simulink model "EEE3099S_Group12_Maze_Sim"  (R2021b)
settings: Solver=FixedStepDiscrete  StartTime=0.0  StopTime=20  FixedStep=0.01  RelTol=1e-3
values from neighbouring files (symbols this model uses):
  axleLength = 0.136    [robotParameters.m]    (also in straight_line.mat = 0.28)
  InputPWM = [-127 -126 -125 -124 -123 -122 -121 -120 -119 -118 -117 -116 ... (173 elements, 1x173)]    [straight_line.mat]
  ticksPerRot = 20    [robotParameters.m]    (also in straight_line.mat)
  wheelR = 0.031    [robotParameters.m]    (also in straight_line.mat = 0.052)
  WheelSpeed = [-12.5105278523 -12.3751973908 -12.2398669292 -12.1045364677 -11.9692060062 -11.8338755446 -11.6985450831 -11.5632146215 -11.42788416 -11.2925536985 -11.1572232369 -11.0218927754 ... (173 elements, 1x173)]    [straight_line.mat]
libraries: mobileRoboticsTrainingLib x6, slpidlib x1, simulink_extras x1
settings Model: ExtModeTrigDuration=2  Creator=Boitumelo  LastModifiedBy=ryanj
settings OptimizationCC: EnhancedBackFolding=on  PassReuseOutputArgsAs=Individual arguments  ZeroExternalMemoryAtStartup=off  ZeroInternalMemoryAtStartup=off  MaxStackSize=64  OptimizeBlockOrder=speed  DifferentSizesBufferReuse=on  OptimizationCustomize=off  EfficientTunableParamExpr=on
settings DebuggingCC: ParameterTunabilityLossMsg=error
settings HardwareCC: ProdBitPerPointer=32  ProdBitPerSizeT=32  ProdBitPerPtrDiffT=32  ProdLargestAtomicInteger=Long  ProdLargestAtomicFloat=Double  ProdWordSize=32  ProdHWDeviceType=ARM Compatible->ARM Cortex  UseEmbeddedCoderFeatures=off  UseSimulinkCoderFeatures=off
settings SFSimCC: MATLABDynamicMemAlloc=off
settings RTWCC: Description=Embedded Coder  SystemTargetFile=ert.tlc  HardwareBoard=Arduino Nano 33 IoT  TemplateMakefile=ert_default_tmf  Toolchain=Arduino ARM
settings CodeAppCC: ForceParamTrailComments=on  IgnoreCustomStorageClasses=off  OperatorAnnotations=on  SimulinkDataObjDesc=on  SFDataObjDesc=on  InsertBlockDesc=on
settings ERTTargetCC: SupportContinuousTime=on  SupportNonInlinedSFcns=on  SupportVariableSizeSignals=on  ExtModeTransport=3  ExtModeStaticAlloc=on  ExtModeStaticAllocSize=8192  ExtModeMexFile=ext_xcp  ExtModeIntrfLevel=Level2 - Open

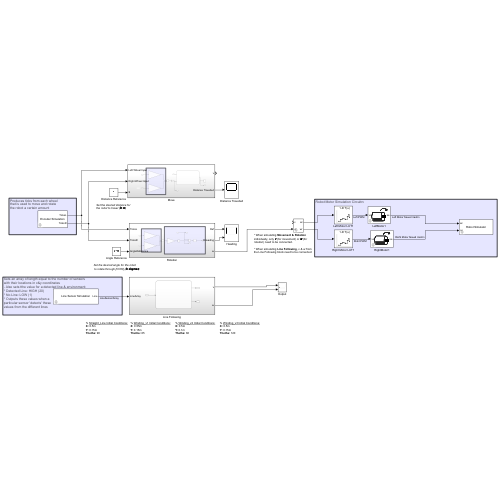
[thumbnail: Simulink's stored preview of the top-level diagram]
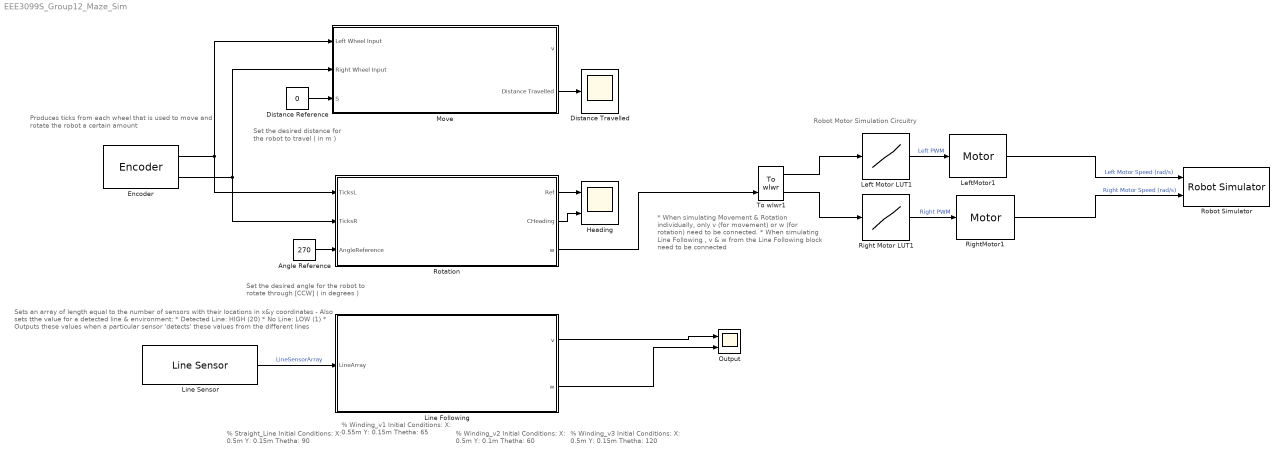
== system EEE3099S_Group12_Maze_Sim ==
  note: * When simulating Movement & Rotation individually, only v (for movement) or w (for rotation) need to be connected.
      |
      | * When simulating Line Following , v & w from the Line Following block need to be connected
  note: % Straight_Line Initial Conditions:
      | X: 0.5m
      | Y: 0.15m
      | Thetha: 90
  note: Sets an array of length equal to the number of sensors
      | with their locations in x&y coordinates
      | - Also sets tthe value for a detected line & environment:
      | * Detected Line: HIGH (20)
      | * No Line: LOW (1)
      | * Outputs these values when a
      | particular sensor 'detects' these
      | values from the different lines
  note: Produces ticks from each wheel
      | that is used to move and rotate
      | the robot a certain amount
  note: Set the desired distance for
      | the robot to travel ( in m )
  note: Robot Motor Simulation Circuitry
  note: Set the desired angle for the robot
      | to rotate through [CCW] ( in degrees )
  note: % Winding_v1 Initial Conditions:
      | X: 0.55m
      | Y: 0.15m
      | Thetha: 65
  note: % Winding_v2 Initial Conditions:
      | X: 0.5m
      | Y: 0.1m
      | Thetha: 60
  note: % Winding_v3 Initial Conditions:
      | X: 0.5m
      | Y: 0.15m
      | Thetha: 120
  Angle Reference : Constant  Value=270
  Distance Reference : Constant  Value=0
  Distance Travelled : Scope
  Encoder : mobileRoboticsTrainingLib/Encoder  axleLength=axleLength  wheelR=wheelR  ticksPerRot=ticksPerRot
      settings: SourceProductName=Mobile Robotics Training Library
  Heading : Scope  NumInputPorts=2
  Left Motor LUT1 : Lookup_n-D  NumberOfTableDimensions=1  BreakpointsForDimension1=WheelSpeed  Table=InputPWM  InterpMethod=Nearest  ExtrapMethod=Clip  InternalRulePriority=Speed  RndMeth=Simplest  InputSameDT=on
  LeftMotor1 : mobileRoboticsTrainingLib/Motor  motorPlant=wheelMotorModel  sensorType=Speed
      settings: SourceProductName=Mobile Robotics Training Library
  Line Following : Subsystem
  Line Sensor : mobileRoboticsTrainingLib/Line Sensor  mapVariable=mapForSim  envVal=1  lineVal=20  sensOff=[0.0643 0.0354; 0.0675 0.005; 0.0675 -0.005; 0.0643 -0.0354]
      settings: SourceProductName=Mobile Robotics Training Library
  Move : Subsystem
  Output : Scope  NumInputPorts=2
  Right Motor LUT1 : Lookup_n-D  NumberOfTableDimensions=1  BreakpointsForDimension1=WheelSpeed  Table=InputPWM  InterpMethod=Nearest  ExtrapMethod=Clip  InternalRulePriority=Speed  RndMeth=Simplest  InputSameDT=on
  RightMotor1 : mobileRoboticsTrainingLib/Motor  motorPlant=wheelMotorModel  sensorType=Speed
      settings: SourceProductName=Mobile Robotics Training Library
  Robot Simulator : mobileRoboticsTrainingLib/Robot Simulator  Priority=99  mapVar=mapForSim  startX=0.5  startY=1  startTheta=0  axleLength=axleLength  wheelR=wheelR
  Rotation : Subsystem
  To wlwr1 : mobileRoboticsTrainingLib/To wlwr  axleLength=0.1  wheelR=0.05
  wires:
  Line Sensor/1 -> Line Following/1(LineArray)  "LineSensorArray"
  Rotation/1(Ref) -> Heading/1
  Rotation/2(CHeading) -> Heading/2
  Angle Reference/1 -> Rotation/3(AngleReference)
  Encoder/1 -> Move/1(Left Wheel Input), Rotation/1(TicksL)
  Encoder/2 -> Move/2(Right Wheel Input), Rotation/2(TicksR)
  Right Motor LUT1/1 -> RightMotor1/1  "Right PWM"
  To wlwr1/1 -> Left Motor LUT1/1
  LeftMotor1/1 -> Robot Simulator/1  "Left Motor Speed (rad/s)"
  RightMotor1/1 -> Robot Simulator/2  "Right Motor Speed (rad/s)"
  To wlwr1/2 -> Right Motor LUT1/1
  Left Motor LUT1/1 -> LeftMotor1/1  "Left PWM"
  Move/2(Distance Travelled) -> Distance Travelled/1
  Distance Reference/1 -> Move/3(S)
  Line Following/1(v) -> Output/1
  Line Following/2(w) -> Output/2
  Rotation/3(w) -> To wlwr1/2

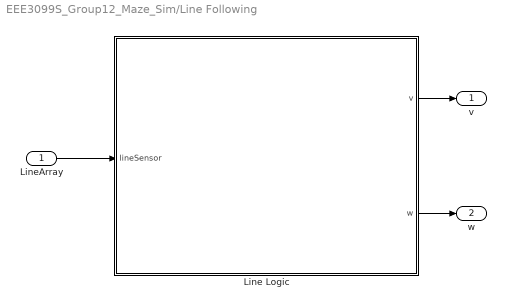
== system EEE3099S_Group12_Maze_Sim/Line Following ==
  LineArray : Inport
  Line Logic : Stateflow chart  TreatAsAtomicUnit=on
  v : Outport
  w : Outport  Port=2
  wires:
  Line Logic/1(v) -> v/1
  Line Logic/2(w) -> w/1
  LineArray/1 -> Line Logic/1(lineSensor)

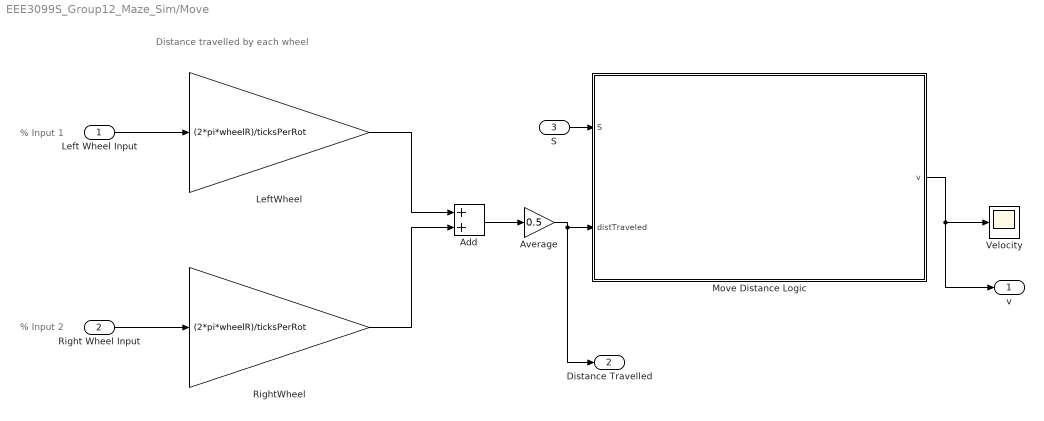
== system EEE3099S_Group12_Maze_Sim/Move ==
  note: Distance travelled by each wheel
  note: % Input 1
  note: % Input 2
  Left Wheel Input : Inport
  Right Wheel Input : Inport  Port=2
  S : Inport  Port=3
  Add : Sum
  Average : Gain  Gain=0.5
  LeftWheel : Gain  Gain=(2*pi*wheelR)/ticksPerRot
  Move Distance Logic : Stateflow chart  TreatAsAtomicUnit=on
  RightWheel : Gain  Gain=(2*pi*wheelR)/ticksPerRot
  Velocity : Scope
  v : Outport
  Distance Travelled : Outport  Port=2
  wires:
  Left Wheel Input/1 -> LeftWheel/1
  LeftWheel/1 -> Add/1
  Right Wheel Input/1 -> RightWheel/1
  S/1 -> Move Distance Logic/1(S)
  Move Distance Logic/1(v) -> v/1, Velocity/1
  RightWheel/1 -> Add/2
  Add/1 -> Average/1
  Average/1 -> Move Distance Logic/2(distTraveled), Distance Travelled/1

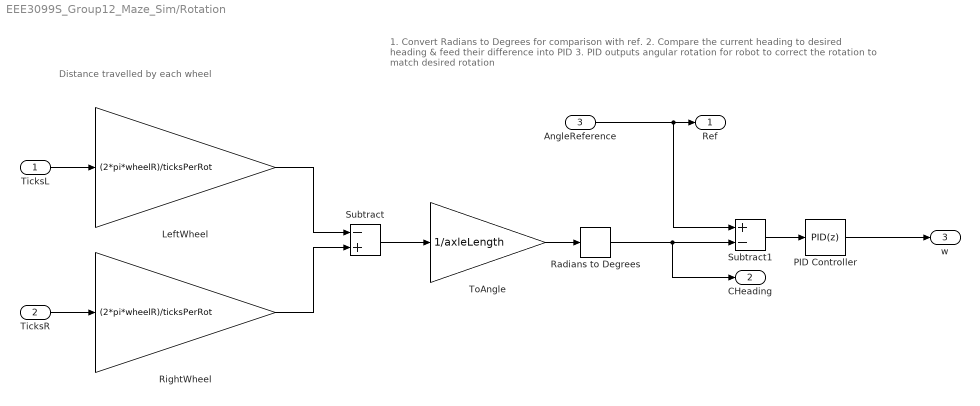
== system EEE3099S_Group12_Maze_Sim/Rotation ==
  note: 1. Convert Radians to Degrees for comparison with ref.
      | 2. Compare the current heading to desired heading
      | & feed their difference into PID
      | 3. PID outputs angular rotation for robot to correct
      | the rotation to match desired rotation
  note: Distance travelled by each wheel
  TicksL : Inport
  TicksR : Inport  Port=2
  AngleReference : Inport  Port=3
  LeftWheel : Gain  Gain=(2*pi*wheelR)/ticksPerRot
  PID Controller : slpidlib/PID Controller  Controller=PID  Form=Parallel  TimeDomain=Discrete-time  UseExternalTs=off  SampleTime=-1  IntegratorMethod=Forward Euler  FilterMethod=Forward Euler  ControllerParametersSource=internal  P=0.111  I=0.001  D=0  UseFilter=off  N=100  TunerSelectOption=Transfer Function Based (PID Tuner App)  InitialConditionSource=internal  InitialConditionForIntegrator=0  InitialConditionForFilter=0  DifferentiatorICPrevScaledInput=0  ExternalReset=none  TrackingMode=off  Kt=1  LimitOutput=on  SatLimitsSource=internal  UpperSaturationLimit=4  LowerSaturationLimit=-4  LinearizeAsGain=on  AntiWindupMode=clamping  Kb=1  POutMin=[]  POutMax=[]  IOutMin=[]  IOutMax=[]  DOutMin=[]  DOutMax=[]  NOutMin=[]  NOutMax=[]  SumOutMin=[]  SumOutMax=[]  SaturationOutMin=[]  SaturationOutMax=[]  PParamMin=[]  PParamMax=[]  IParamMin=[]  IParamMax=[]  DParamMin=[]  DParamMax=[]  NParamMin=[]  NParamMax=[]  KbParamMin=[]  KbParamMax=[]  KtParamMin=[]  KtParamMax=[]  KbOutMin=[]  KbOutMax=[]  KtOutMin=[]  KtOutMax=[]  IntegratorOutMin=[]  IntegratorOutMax=[]  FilterOutMin=[]  FilterOutMax=[]  SumI1OutMin=[]  SumI1OutMax=[]  SumI2OutMin=[]  SumI2OutMax=[]  SumI3OutMin=[]  SumI3OutMax=[]  SumI4OutMin=[]  SumI4OutMax=[]  SumDOutMin=[]  SumDOutMax=[]  DifferentiatorOutMin=[]  DifferentiatorOutMax=[]  FilterDiffOutCoefMin=[]  FilterDiffOutCoefMax=[]  ReciprocalOutMin=[]  ReciprocalOutMax=[]  SumDenOutMin=[]  SumDenOutMax=[]  SumNumOutMin=[]  SumNumOutMax=[]  DivideOutMin=[]  DivideOutMax=[]  UdiffTsProdOutMin=[]  UdiffTsProdOutMax=[]  NTsProdOutMin=[]  NTsProdOutMax=[]  UintegralTsProdOutMin=[]  UintegralTsProdOutMax=[]  UngainTsProdOutMin=[]  UngainTsProdOutMax=[]  IntegratorContinuousStateAttributes=''  IntegratorStateMustResolveToSignalObject=off  IntegratorRTWStateStorageClass=Auto  FilterContinuousStateAttributes=''  FilterStateMustResolveToSignalObject=off  FilterRTWStateStorageClass=Auto  ParallelPVariant=InternalParameters  IdealPVariant=Disabled  IVariant=InternalParameters  DVariant=InternalParameters  IntegratorVariant=Discrete  SatVariant=Enabled  AWVariant=DiscClampingParallel  PCopyVariant=Disabled  TRVariant=Disabled  FdbkBlocksVariant=Forward  IdealPFdbkVariant=Disabled  SatFdbkVariant=Disabled  DerivativeFilterVariant=Differentiator  NVariant=Passthrough  NCopyVariant=Disabled_SignalSpec  FilterICVariant=InternalICsDifferentiator  IntegratorICVariant=InternalICs  ExternalResetVariant=Disabled  TRSumVariant=Passthrough  SumFdbkVariant=Disabled  SumVariant=Sum_PID  TsampFilterVariant=InternalTs  TsampNgainVariant=Passthrough  TsampIntegralVariant=Passthrough  ExternalSaturationOutDataTypeStr=Inherit: Same as second input  InitialConditionSetting=Output
  Radians to Degrees : simulink_extras/Transformations/Radians to Degrees
  RightWheel : Gain  Gain=(2*pi*wheelR)/ticksPerRot
  Subtract : Sum  Inputs=-+
  Subtract1 : Sum  Inputs=+-
  ToAngle : Gain  Gain=1/axleLength
  Ref : Outport
  CHeading : Outport  Port=2
  w : Outport  Port=3
  wires:
  RightWheel/1 -> Subtract/2
  LeftWheel/1 -> Subtract/1
  Subtract/1 -> ToAngle/1
  Subtract1/1 -> PID Controller/1
  Radians to Degrees/1 -> CHeading/1, Subtract1/2
  AngleReference/1 -> Ref/1, Subtract1/1
  TicksL/1 -> LeftWheel/1
  ToAngle/1 -> Radians to Degrees/1
  TicksR/1 -> RightWheel/1
  PID Controller/1 -> w/1

== stateflow chart EEE3099S_Group12_Maze_Sim/Line Following/Line Logic ==
  state FollowLine
    state Straight
      entry:
      v=0.035;
      w=0;
    note: % If LHS, middle sensor doesn't detect a line, correct this by bearing right
    note: % If RHS, middle sensor doesn't detect a line, correct this by bearing left
    state BearRight
      entry:
      w=-0.2;
    state BearLeft
      entry:
      w=0.2;
    (default) -> Straight
    Straight -> BearRight [order 2] : [lineSensor(2)<10]
    Straight -> BearLeft [order 1] : [lineSensor(3)<10]
    BearRight -> Straight : [lineSensor(3)>=10 && lineSensor(2)>=10]
    BearLeft -> Straight : [lineSensor(3)>=10 && lineSensor(2)>=10]
  note: % Both middle sensors detect a line, and the robot can continue going straight
  (default) -> FollowLine : % Line Following Logic States
  data: v output; w output; lineSensor input

== stateflow chart EEE3099S_Group12_Maze_Sim/Move/Move Distance Logic ==
  state MoveForward
    entry:
    v = 0.1;
  note: % Sets robot to move forward @ v=0.1 m/s
  state Stop
    entry:
    v = 0;
  note: % Sets the velocity of the robot to 0 m/s when the desired distance has been travelled
  (default) -> MoveForward : %Start Move Distance
  MoveForward -> Stop : [distTraveled >= S]
  data: S input; v output; distTraveled input
